simulink model "SpaceFlexibleRobotAug"  (R2025b)
settings: Solver=VariableStepAuto  StartTime=0.0  StopTime=10.0  RelTol=1e-3
undefined symbols (not defined in the file): Ignew, InvDyn, InvDynAug, Jr, ra_norm, sig4, ureal, uss
libraries: RCTblocks x133, SDTlibV2 x4
(part 3 of 3)

== system SpaceFlexibleRobotAug/link 6/Revolute joint + configuration/18x18 v-u_rotation/Subsystem2 ==
  In1 : Inport
  Demux : Demux  Outputs=3
  Gain : Gain  Gain=2
  Gain1 : Gain  Gain=-2
  Gain2 : Gain  Gain=2
  Gain3 : Gain  Gain=2
  Gain4 : Gain  Gain=pass  Multiplication=Matrix(K*u) (u vector)
  Gain5 : Gain  Gain=pass'  Multiplication=Matrix(K*u) (u vector)
  Mux : Mux  Inputs=3
  Sum : Sum  Inputs=++|
  Sum1 : Sum  Inputs=|++
  Sum2 : Sum  Inputs=|+-
  Sum3 : Sum  Inputs=|++
  Sum4 : Sum  Inputs=++|
  Sum5 : Sum  Inputs=++|
  Uncertain State Space{,1..3} (4 alike) : RCTblocks/Uncertain State Space  Tag=USS  USystem=uss(sig4)  UValue=[]  X0=[]  uX0=[]
  Out1 : Outport  VectorParamsAs1DForOutWhenUnconnected=off
  wires:
  Sum5/1 -> Gain2/1
  Sum1/1 -> Mux/1
  Sum2/1 -> Gain/1
  Uncertain State Space1/1 -> Sum/1
  Demux/2 -> Gain1/1, Sum4/1
  Sum/1 -> Uncertain State Space/1
  Gain3/1 -> Sum5/2
  Uncertain State Space/1 -> Sum1/1, Sum5/1, Uncertain State Space1/1
  Gain1/1 -> Sum2/1
  Sum3/1 -> Uncertain State Space2/1
  Sum4/1 -> Mux/2
  Mux/1 -> Gain4/1
  Demux/3 -> Mux/3
  Demux/1 -> Sum1/2, Gain3/1
  Uncertain State Space2/1 -> Sum2/2, Sum4/2, Uncertain State Space3/1
  Gain/1 -> Sum/2
  In1/1 -> Gain5/1
  Gain2/1 -> Sum3/1
  Uncertain State Space3/1 -> Sum3/2
  Gain4/1 -> Out1/1
  Gain5/1 -> Demux/1

== system SpaceFlexibleRobotAug/link 6/Revolute joint + configuration/18x18 v-u_rotation/Subsystem3 ==
  In1 : Inport
  Demux : Demux  Outputs=3
  Gain : Gain  Gain=2
  Gain1 : Gain  Gain=-2
  Gain2 : Gain  Gain=2
  Gain3 : Gain  Gain=2
  Gain4 : Gain  Gain=pass  Multiplication=Matrix(K*u) (u vector)
  Gain5 : Gain  Gain=pass'  Multiplication=Matrix(K*u) (u vector)
  Mux : Mux  Inputs=3
  Sum : Sum  Inputs=++|
  Sum1 : Sum  Inputs=|++
  Sum2 : Sum  Inputs=|+-
  Sum3 : Sum  Inputs=|++
  Sum4 : Sum  Inputs=++|
  Sum5 : Sum  Inputs=++|
  Uncertain State Space{,1..3} (4 alike) : RCTblocks/Uncertain State Space  Tag=USS  USystem=uss(sig4)  UValue=[]  X0=[]  uX0=[]
  Out1 : Outport  VectorParamsAs1DForOutWhenUnconnected=off
  wires:
  Gain4/1 -> Out1/1
  Uncertain State Space3/1 -> Sum3/2
  Gain2/1 -> Sum3/1
  In1/1 -> Gain5/1
  Gain/1 -> Sum/2
  Uncertain State Space2/1 -> Uncertain State Space3/1, Sum4/2, Sum2/2
  Demux/1 -> Gain3/1, Sum1/2
  Demux/3 -> Mux/3
  Mux/1 -> Gain4/1
  Sum4/1 -> Mux/2
  Sum3/1 -> Uncertain State Space2/1
  Gain1/1 -> Sum2/1
  Uncertain State Space/1 -> Uncertain State Space1/1, Sum5/1, Sum1/1
  Gain3/1 -> Sum5/2
  Sum/1 -> Uncertain State Space/1
  Demux/2 -> Sum4/1, Gain1/1
  Uncertain State Space1/1 -> Sum/1
  Sum2/1 -> Gain/1
  Sum1/1 -> Mux/1
  Sum5/1 -> Gain2/1
  Gain5/1 -> Demux/1

== system SpaceFlexibleRobotAug/link 6/Revolute joint + configuration/18x18 v-u_rotation/Subsystem4 ==
  In1 : Inport
  Demux : Demux  Outputs=3
  Gain : Gain  Gain=2
  Gain1 : Gain  Gain=-2
  Gain2 : Gain  Gain=2
  Gain3 : Gain  Gain=2
  Gain4 : Gain  Gain=pass  Multiplication=Matrix(K*u) (u vector)
  Gain5 : Gain  Gain=pass'  Multiplication=Matrix(K*u) (u vector)
  Mux : Mux  Inputs=3
  Sum : Sum  Inputs=++|
  Sum1 : Sum  Inputs=|++
  Sum2 : Sum  Inputs=|+-
  Sum3 : Sum  Inputs=|++
  Sum4 : Sum  Inputs=++|
  Sum5 : Sum  Inputs=++|
  Uncertain State Space{,1..3} (4 alike) : RCTblocks/Uncertain State Space  Tag=USS  USystem=uss(sig4)  UValue=[]  X0=[]  uX0=[]
  Out1 : Outport  VectorParamsAs1DForOutWhenUnconnected=off
  wires:
  Gain5/1 -> Demux/1
  Gain4/1 -> Out1/1
  Uncertain State Space3/1 -> Sum3/2
  Gain2/1 -> Sum3/1
  In1/1 -> Gain5/1
  Gain/1 -> Sum/2
  Uncertain State Space2/1 -> Uncertain State Space3/1, Sum4/2, Sum2/2
  Demux/1 -> Gain3/1, Sum1/2
  Demux/3 -> Mux/3
  Mux/1 -> Gain4/1
  Sum4/1 -> Mux/2
  Sum3/1 -> Uncertain State Space2/1
  Gain1/1 -> Sum2/1
  Uncertain State Space/1 -> Uncertain State Space1/1, Sum5/1, Sum1/1
  Gain3/1 -> Sum5/2
  Sum/1 -> Uncertain State Space/1
  Demux/2 -> Sum4/1, Gain1/1
  Uncertain State Space1/1 -> Sum/1
  Sum2/1 -> Gain/1
  Sum1/1 -> Mux/1
  Sum5/1 -> Gain2/1

== system SpaceFlexibleRobotAug/link 6/Revolute joint + configuration/18x18 v-u_rotation/Subsystem5 ==
  In1 : Inport
  Demux : Demux  Outputs=3
  Gain : Gain  Gain=2
  Gain1 : Gain  Gain=-2
  Gain2 : Gain  Gain=2
  Gain3 : Gain  Gain=2
  Gain4 : Gain  Gain=pass  Multiplication=Matrix(K*u) (u vector)
  Gain5 : Gain  Gain=pass'  Multiplication=Matrix(K*u) (u vector)
  Mux : Mux  Inputs=3
  Sum : Sum  Inputs=++|
  Sum1 : Sum  Inputs=|++
  Sum2 : Sum  Inputs=|+-
  Sum3 : Sum  Inputs=|++
  Sum4 : Sum  Inputs=++|
  Sum5 : Sum  Inputs=++|
  Uncertain State Space{,1..3} (4 alike) : RCTblocks/Uncertain State Space  Tag=USS  USystem=uss(sig4)  UValue=[]  X0=[]  uX0=[]
  Out1 : Outport  VectorParamsAs1DForOutWhenUnconnected=off
  wires:
  Gain5/1 -> Demux/1
  Sum5/1 -> Gain2/1
  Sum1/1 -> Mux/1
  Sum2/1 -> Gain/1
  Uncertain State Space1/1 -> Sum/1
  Demux/2 -> Gain1/1, Sum4/1
  Sum/1 -> Uncertain State Space/1
  Gain3/1 -> Sum5/2
  Uncertain State Space/1 -> Sum1/1, Sum5/1, Uncertain State Space1/1
  Gain1/1 -> Sum2/1
  Sum3/1 -> Uncertain State Space2/1
  Sum4/1 -> Mux/2
  Mux/1 -> Gain4/1
  Demux/3 -> Mux/3
  Demux/1 -> Sum1/2, Gain3/1
  Uncertain State Space2/1 -> Sum2/2, Sum4/2, Uncertain State Space3/1
  Gain/1 -> Sum/2
  In1/1 -> Gain5/1
  Gain2/1 -> Sum3/1
  Uncertain State Space3/1 -> Sum3/2
  Gain4/1 -> Out1/1

== system SpaceFlexibleRobotAug/link 6/Revolute joint + configuration/6x6 v-u_rotation/Subsystem ==
  In1 : Inport
  Demux : Demux  Outputs=3
  Gain : Gain  Gain=2
  Gain1 : Gain  Gain=-2
  Gain2 : Gain  Gain=2
  Gain3 : Gain  Gain=2
  Gain4 : Gain  Gain=pass  Multiplication=Matrix(K*u) (u vector)
  Gain9 : Gain  Gain=pass'  Multiplication=Matrix(K*u) (u vector)
  Mux : Mux  Inputs=3
  Sum : Sum  Inputs=++|
  Sum1 : Sum  Inputs=|++
  Sum2 : Sum  Inputs=|+-
  Sum3 : Sum  Inputs=|++
  Sum4 : Sum  Inputs=++|
  Sum5 : Sum  Inputs=++|
  Uncertain State Space{,1..3} (4 alike) : RCTblocks/Uncertain State Space  Tag=USS  USystem=uss(sig4)  UValue=[]  X0=[]  uX0=[]
  Out1 : Outport  VectorParamsAs1DForOutWhenUnconnected=off
  wires:
  Sum5/1 -> Gain2/1
  Sum1/1 -> Mux/1
  Sum2/1 -> Gain/1
  Uncertain State Space1/1 -> Sum/1
  Demux/2 -> Gain1/1, Sum4/1
  Sum/1 -> Uncertain State Space/1
  Gain3/1 -> Sum5/2
  Uncertain State Space/1 -> Sum1/1, Sum5/1, Uncertain State Space1/1
  Gain1/1 -> Sum2/1
  Sum3/1 -> Uncertain State Space2/1
  Sum4/1 -> Mux/2
  In1/1 -> Gain9/1
  Mux/1 -> Gain4/1
  Demux/3 -> Mux/3
  Demux/1 -> Sum1/2, Gain3/1
  Uncertain State Space2/1 -> Sum2/2, Sum4/2, Uncertain State Space3/1
  Gain/1 -> Sum/2
  Gain9/1 -> Demux/1
  Gain2/1 -> Sum3/1
  Uncertain State Space3/1 -> Sum3/2
  Gain4/1 -> Out1/1

== system SpaceFlexibleRobotAug/link 6/Revolute joint + configuration/6x6 v-u_rotation/Subsystem1 ==
  In1 : Inport
  Demux : Demux  Outputs=3
  Gain : Gain  Gain=2
  Gain1 : Gain  Gain=-2
  Gain2 : Gain  Gain=2
  Gain3 : Gain  Gain=2
  Gain4 : Gain  Gain=pass  Multiplication=Matrix(K*u) (u vector)
  Gain9 : Gain  Gain=pass'  Multiplication=Matrix(K*u) (u vector)
  Mux : Mux  Inputs=3
  Sum : Sum  Inputs=++|
  Sum1 : Sum  Inputs=|++
  Sum2 : Sum  Inputs=|+-
  Sum3 : Sum  Inputs=|++
  Sum4 : Sum  Inputs=++|
  Sum5 : Sum  Inputs=++|
  Uncertain State Space{,1..3} (4 alike) : RCTblocks/Uncertain State Space  Tag=USS  USystem=uss(sig4)  UValue=[]  X0=[]  uX0=[]
  Out1 : Outport  VectorParamsAs1DForOutWhenUnconnected=off
  wires:
  Gain4/1 -> Out1/1
  Uncertain State Space3/1 -> Sum3/2
  Gain2/1 -> Sum3/1
  Gain9/1 -> Demux/1
  Gain/1 -> Sum/2
  Uncertain State Space2/1 -> Uncertain State Space3/1, Sum4/2, Sum2/2
  Demux/1 -> Gain3/1, Sum1/2
  Demux/3 -> Mux/3
  Mux/1 -> Gain4/1
  In1/1 -> Gain9/1
  Sum4/1 -> Mux/2
  Sum3/1 -> Uncertain State Space2/1
  Gain1/1 -> Sum2/1
  Uncertain State Space/1 -> Uncertain State Space1/1, Sum5/1, Sum1/1
  Gain3/1 -> Sum5/2
  Sum/1 -> Uncertain State Space/1
  Demux/2 -> Sum4/1, Gain1/1
  Uncertain State Space1/1 -> Sum/1
  Sum2/1 -> Gain/1
  Sum1/1 -> Mux/1
  Sum5/1 -> Gain2/1
